simulink model "exemple4"  (R2021a)
settings: Solver=FixedStepDiscrete  StartTime=0.0  StopTime=0.1  RelTol=1e-3  EnableMultiTasking=on
values from neighbouring files (symbols this model uses):
  rep = reshape(a', 13*Ns, 1)'    [CalculREP.m]
  user = 1    [Launch_Sync.m]
libraries: dspsrcs4 x7, simulink x5, commfilt2 x4, dspsigops x3, dspswit3 x3, dspindex x2, commutil2 x1, simulink_extras x1
settings Model: Creator=sebastienroy  LastModifiedBy=antho
settings SolverCC: AlgebraicLoopSolver=TrustRegion
settings DataIOCC: InitialState=mod  LimitDataPoints=on  SaveFormat=Array  ReturnWorkspaceOutputs=off
settings OptimizationCC: LifeSpan=inf
settings DebuggingCC: UnderspecifiedInitializationDetection=Classic  MergeDetectMultiDrivingBlocksExec=none  SolverPrmCheckMsg=warning  StateNameClashWarn=warning  SFUnexpectedBacktrackingDiag=warning  SFNoUnconditionalDefaultTransitionDiag=warning  SFExecutionAtInitializationDiag=none  SFMachineParentedDataDiag=warning  ArithmeticOperatorsInVariantConditions=warning
settings HardwareCC: ProdBitPerPointer=32  ProdBitPerSizeT=32  ProdBitPerPtrDiffT=32  ProdLargestAtomicFloat=None  ProdIntDivRoundTo=Undefined  ProdEndianess=Unspecified  ProdWordSize=32  ProdHWDeviceType=32-bit Generic
settings ModelReferenceCC: PropagateSignalLabelsOutOfModel=off
settings SFSimCC: SimUseLocalCustomCode=off  CustomCodeUndefinedFunction=UseInterfaceOnly
settings RTWCC: RTWUseLocalCustomCode=off
settings CodeAppCC: StateflowObjectComments=on
settings GRTTargetCC: TargetLangStandard=C89/C90 (ANSI)
settings ConfigComp: CovMetricSettings=dw  CovSaveCumulativeToWorkspaceVar=on  CovSaveSingleToWorkspaceVar=on  CovExternalEMLEnable=off
settings SimscapeCC: SimscapeNormalizeSystem=off
settings ConfigurationSet: Description=SimMechanics 2G

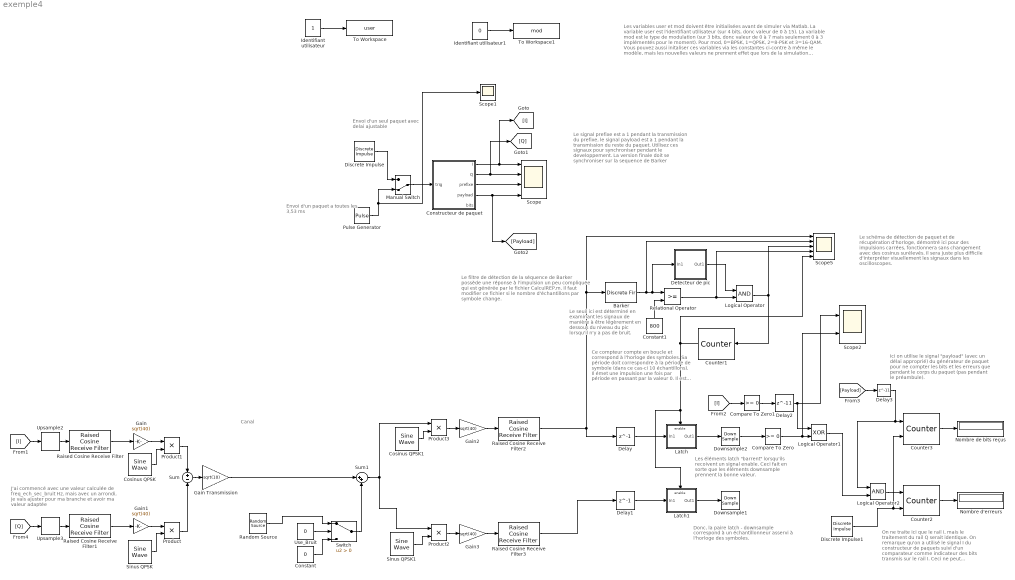
== system exemple4 ==
  note: Le filtre de détection de la séquence de Barker
      | possède une réponse à l'impulsion un peu
      | compliquée qui est générée par le fichier
      | CalculREP.m. Il faut modifier ce fichier si le nombre
      | d'échantillons par symbole change.
  note: Le schéma de détection de paquet et
      | de récupération d'horloge, démontré ici
      | pour des impulsions carrées, fonctionnera
      | sans changement avec des cosinus surélevés.
      | Il sera juste plus difficile d'interpréter visuellement
      | les signaux dans les oscilloscopes.
  note: On ne traite ici que le rail I, mais le
      | traitement du rail Q serait identique.
      | On remarque qu'on a utilisé le signal
      | I du constructeur de paquets suivi
      | d'un comparateur comme indicateur
      | des bits transmis sur le rail I. Ceci ne
      | peut fonctionner qu'en BPSK ou QPSK.
      | Dans le cas général, il faudrait utiliser la
      | sortie "bits" du générateur.
  note: Ici on utilise le signal "payload" (avec
      | un délai approprié) du générateur de
      | paquet pour ne compter les bits et les
      | erreurs que pendant le corps du paquet
      |  (pas pendant le préambule).
  note: Donc, la paire latch - downsample
      | correspond à un échantillonneur asservi
      | à l'horloge des symboles.
  note: Les éléments latch "barrent"
      | lorsqu'ils recoivent un signal enable.
      | Ceci fait en sorte que les éléments
      | downsample prennent la bonne valeur.
  note: Le seuil ici est déterminé
      | en examinant les signaux
      | de manière à être légèrement
      | en dessous du niveau du pic
      | lorsqu'il n'y a pas de bruit.
  note: Ce compteur compte en boucle et
      | correspond à l'horloge des symboles.
      | Sa période doit correspondre à
      | la période de symbole (dans ce
      | cas-ci 10 échantillons). Il émet
      | une impulsion une fois par
      | période en passant par la
      | valeur 0. Il est remis à zéro par
      | le pic de détection de début de paquet.
  note: Le signal prefixe est a 1 pendant
      | la transmission du prefixe, le signal payload
      | est a 1 pendant la transmission du reste du
      | paquet. Utilisez ces signaux pour synchroniser
      | pendant le developpement. La version finale
      | doit se synchroniser sur la sequence de Barker
  note: Les variables user et mod doivent être initialisées avant
      | de simuler via Matlab.
      | La variable user est l'identifiant utilisateur (sur 4 bits, donc valeur de 0 à 15).
      |
      | La variable mod est le type de modulation (sur 3 bits, donc valeur de 0 à 7
      | mais seulement 0 à 3 implémentés pour le moment). Pour mod, 0=BPSK,
      | 1=QPSK, 2=8-PSK et 3=16-QAM.
      |
      | Vous pouvez aussi initaliser ces variables via les constantes ci-contre à même
      | le modèle, mais les nouvelles valeurs ne prennent effet que lors de la simulation
      | suivante.
      |
      | Ces variables sont automatiquement incluses dans le préambule du paquet.
  note: Envoi d'un paquet
      | a toutes les 3,53 ms
  note: Envoi d'un seul
      | paquet avec delai
      | ajustable
  note: Canal
  note: J'ai commencé avec une valeur calculée de freq_ech_sec_bruit Hz, mais avec un arrondi, je vais ajuster pour ma branche et avoir ma valeur adaptée
  Barker : DiscreteFir  Coefficients=rep
  Compare To Zero : simulink/Logic and Bit Operations/Compare To Zero  relop=>=  OutDataTypeStr=boolean
  Compare To Zero1 : simulink/Logic and Bit Operations/Compare To Zero  relop=>=  OutDataTypeStr=boolean
  Constant : Constant  Value=0
  Constant1 : Constant  Value=800  SampleTime=-1
  Constructeur de paquet : Subsystem
  Cosinus QPSK : dspsrcs4/Sine Wave  Amplitude=1  Frequency=1.36e6  Phase=pi/2  SampleMode=Discrete  OutComplex=Real  CompMethod=Trigonometric fcn  TableSize=Speed  SampleTime=1/3400000  SamplesPerFrame=1  ResetState=Restart at time zero  OutputFrames=off  dataType=double  wordLen=16  udDataType=sfix(16)  fracBitsMode=Best precision  numFracBits=15  OutDataTypeStr=double  LastOutDataTypeStr=double
      settings: AttributesFormatString=|
      | Amplitude %<Amplitude>
      | Fréquence %<Frequency>
      | Phase %<Phase>
      | Sample Time %<SampleTime>
  Cosinus QPSK1 : dspsrcs4/Sine Wave  Amplitude=1  Frequency=1.36e6  Phase=pi/2  SampleMode=Discrete  OutComplex=Real  CompMethod=Trigonometric fcn  TableSize=Speed  SampleTime=1/3400000  SamplesPerFrame=1  ResetState=Restart at time zero  OutputFrames=off  dataType=double  wordLen=16  udDataType=sfix(16)  fracBitsMode=Best precision  numFracBits=15  OutDataTypeStr=double  LastOutDataTypeStr=double
      settings: AttributesFormatString=|
      | Amplitude %<Amplitude>
      | Fréquence %<Frequency>
      | Phase %<Phase>
      | Sample Time %<SampleTime>
  Counter1 : dspswit3/Counter  Direction=Up  CountEvent=Free running  CounterSize=User defined  MaxCount=9  InitialCount=0  Output=Hit  HitValue=0  ResetInput=on  SamplesPerFrame=1  Ts=-1  CntDtype=double  HitDtype=Logical
  Counter2 : dspswit3/Counter  Direction=Up  CountEvent=Non-zero sample  CounterSize=32 bits  MaxCount=255  InitialCount=0  Output=Count  HitValue=32  ResetInput=on  SamplesPerFrame=1  Ts=1/10000  CntDtype=double  HitDtype=Logical
  Counter3 : dspswit3/Counter  Direction=Up  CountEvent=Non-zero sample  CounterSize=32 bits  MaxCount=255  InitialCount=0  Output=Count  HitValue=32  ResetInput=on  SamplesPerFrame=1  Ts=1/10000  CntDtype=double  HitDtype=Logical
  Delay : Delay  DelayLength=1  InitialCondition=0
  Delay1 : Delay  DelayLength=1  InitialCondition=0
  Delay2 : Delay  DelayLength=11  InitialCondition=0
  Delay3 : Delay  DelayLength=11  InitialCondition=0
  Detecteur de pic : Subsystem
  Discrete Impulse : dspsrcs4/Discrete  Impulse  Delay=5  SampleTime=1/85000  FrameSample=1  OutputFrames=on  dataType=double  isSigned=on  wordLen=16  udDataType=sfix(16)  fracBitsMode=Best precision  numFracBits=15  OutDataTypeStr=double  LastOutDataTypeStr=double
  Discrete Impulse1 : dspsrcs4/Discrete  Impulse  Delay=6  SampleTime=1/85000  FrameSample=1  OutputFrames=on  dataType=double  isSigned=on  wordLen=16  udDataType=sfix(16)  fracBitsMode=Best precision  numFracBits=15  OutDataTypeStr=double  LastOutDataTypeStr=double
  Downsample1 : DownSample  N=40  RateOptions=Allow multirate processing
  Downsample2 : DownSample  N=40  RateOptions=Allow multirate processing
  Gain{,1..3} (4 alike) : Gain  Gain=sqrt(40)
  Gain Transmission : Gain  Gain=sqrt(10)
  Identifiant utilisateur : Constant  VectorParams1D=off
  Identifiant utilisateur1 : Constant  Value=0  VectorParams1D=off
  Latch : Subsystem  TreatAsAtomicUnit=on
  Latch1 : Subsystem  TreatAsAtomicUnit=on
  Logical Operator : Logic  AllPortsSameDT=off  OutDataTypeStr=boolean
  Logical Operator1 : Logic  Operator=XOR  AllPortsSameDT=off  OutDataTypeStr=boolean
  Logical Operator2 : Logic  AllPortsSameDT=off  OutDataTypeStr=boolean
  Manual Switch : ManualSwitch  CurrentSetting=0
  Nombre d'erreurs : Display
  Nombre de bits reçus : Display
  Product{,1..3} (4 alike) : Product
  Pulse Generator : DiscretePulseGenerator  Period=300  SampleTime=1/85000
  Raised Cosine Receive Filter : commfilt2/Raised Cosine Receive Filter  filtType=Square root  R=0.12  filtSpan=10  N=40  downFactor=1  downOffset=0  filterGain=1  RateOptions=Allow multirate processing  framing=Mute  checkCoeff=off  variableName=rcRxFilt  currentFiltSpan=10  D=5  inputOffset=0  sampMode=Mute  saveAsFlag=0  rateMode=Downsampling  checkGain=Normalized  launchFVT=on  roundingMode=Floor  overflowMode=off  coeffDataTypeStr=Inherit: Same word length as input  coeffMin=[]  coeffMax=[]  coeffLastDataTypeStr=Inherit: Same word length as input  accumDataTypeStr=Inherit: Same as product output  accumLastDataTypeStr=Inherit: Same as product output  outputDataTypeStr=Inherit: Same as accumulator  outputMin=[]  outputMax=[]  outputLastDataTypeStr=Inherit: Same as accumulator
      settings: AttributesFormatString=|
      | Type : %<filtType>
      | r : %<R>
      | Span in symb : %<filtSpan>
      | Gain : %<filterGain>
      | Input Samples per symb : 40
  Raised Cosine Receive Filter1 : commfilt2/Raised Cosine Receive Filter  filtType=Square root  R=0.12  filtSpan=10  N=40  downFactor=1  downOffset=0  filterGain=1  RateOptions=Allow multirate processing  framing=Mute  checkCoeff=off  variableName=rcRxFilt1  currentFiltSpan=10  D=5  inputOffset=0  sampMode=Mute  saveAsFlag=0  rateMode=Downsampling  checkGain=Normalized  launchFVT=on  roundingMode=Floor  overflowMode=off  coeffDataTypeStr=Inherit: Same word length as input  coeffMin=[]  coeffMax=[]  coeffLastDataTypeStr=Inherit: Same word length as input  accumDataTypeStr=Inherit: Same as product output  accumLastDataTypeStr=Inherit: Same as product output  outputDataTypeStr=Inherit: Same as accumulator  outputMin=[]  outputMax=[]  outputLastDataTypeStr=Inherit: Same as accumulator
      settings: AttributesFormatString=|
      | Type : %<filtType>
      | r : %<R>
      | Span in symb : %<filtSpan>
      | Gain : %<filterGain>
      | Input Samples per symb : 40
  Raised Cosine Receive Filter2 : commfilt2/Raised Cosine Receive Filter  filtType=Square root  R=0.12  filtSpan=10  N=40  downFactor=1  downOffset=0  filterGain=1  RateOptions=Allow multirate processing  framing=Mute  checkCoeff=off  variableName=rcRxFilt2  currentFiltSpan=10  D=5  inputOffset=0  sampMode=Mute  saveAsFlag=0  rateMode=Downsampling  checkGain=Normalized  launchFVT=on  roundingMode=Floor  overflowMode=off  coeffDataTypeStr=Inherit: Same word length as input  coeffMin=[]  coeffMax=[]  coeffLastDataTypeStr=Inherit: Same word length as input  accumDataTypeStr=Inherit: Same as product output  accumLastDataTypeStr=Inherit: Same as product output  outputDataTypeStr=Inherit: Same as accumulator  outputMin=[]  outputMax=[]  outputLastDataTypeStr=Inherit: Same as accumulator
      settings: AttributesFormatString=|
      | Type : %<filtType>
      | r : %<R>
      | Span in symb : %<filtSpan>
      | Gain : %<filterGain>
      | Input Samples per symb : 40
  Raised Cosine Receive Filter3 : commfilt2/Raised Cosine Receive Filter  filtType=Square root  R=0.12  filtSpan=10  N=40  downFactor=1  downOffset=0  filterGain=1  RateOptions=Allow multirate processing  framing=Mute  checkCoeff=off  variableName=rcRxFilt3  currentFiltSpan=10  D=5  inputOffset=0  sampMode=Mute  saveAsFlag=0  rateMode=Downsampling  checkGain=Normalized  launchFVT=on  roundingMode=Floor  overflowMode=off  coeffDataTypeStr=Inherit: Same word length as input  coeffMin=[]  coeffMax=[]  coeffLastDataTypeStr=Inherit: Same word length as input  accumDataTypeStr=Inherit: Same as product output  accumLastDataTypeStr=Inherit: Same as product output  outputDataTypeStr=Inherit: Same as accumulator  outputMin=[]  outputMax=[]  outputLastDataTypeStr=Inherit: Same as accumulator
      settings: AttributesFormatString=|
      | Type : %<filtType>
      | r : %<R>
      | Span in symb : %<filtSpan>
      | Gain : %<filterGain>
      | Input Samples per symb : 40
  Random Source : dspsrcs4/Random Source  SrcType=Gaussian  NormMethod=Ziggurat  CltLength=12  MinVal=0  MaxVal=1  MeanVal=0  VarVal=37.8072  RepMode=Not repeatable  rawSeed=1  IsInherit=off  SampMode=Discrete  SampTime=1/3.4e6  SampFrame=1  DataType=Double  OutComplex=Real  OutputFrames=off
      settings: AttributesFormatString=|
      | Sample Rate : 1/3.4e6 Hz
      | Variance : 37.8072 W
  Relational Operator : RelationalOperator  OutDataTypeStr=boolean  RndMeth=Nearest
  Scope : Scope  NumInputPorts=4
  Scope1 : Scope
  Scope2 : Scope  NumInputPorts=2
  Scope5 : Scope  NumInputPorts=5
  Sinus QPSK : dspsrcs4/Sine Wave  Amplitude=1  Frequency=1.36e6  Phase=0  SampleMode=Discrete  OutComplex=Real  CompMethod=Trigonometric fcn  TableSize=Speed  SampleTime=1/3400000  SamplesPerFrame=1  ResetState=Restart at time zero  OutputFrames=off  dataType=double  wordLen=16  udDataType=sfix(16)  fracBitsMode=Best precision  numFracBits=15  OutDataTypeStr=double  LastOutDataTypeStr=double
      settings: AttributesFormatString=|
      | Amplitude %<Amplitude>
      | Fréquence %<Frequency>
      | Phase %<Phase>
      | Sample Time %<SampleTime>
  Sinus QPSK1 : dspsrcs4/Sine Wave  Amplitude=-1  Frequency=1.36e6  Phase=0  SampleMode=Discrete  OutComplex=Real  CompMethod=Trigonometric fcn  TableSize=Speed  SampleTime=1/3400000  SamplesPerFrame=1  ResetState=Restart at time zero  OutputFrames=off  dataType=double  wordLen=16  udDataType=sfix(16)  fracBitsMode=Best precision  numFracBits=15  OutDataTypeStr=double  LastOutDataTypeStr=double
      settings: AttributesFormatString=|
      | Amplitude %<Amplitude>
      | Fréquence %<Frequency>
      | Phase %<Phase>
      | Sample Time %<SampleTime>
  Sum : Sum  Inputs=+|-
  Sum1 : Sum  Inputs=|++
  Switch : Switch  Criteria=u2 > Threshold
  To Workspace : ToWorkspace  VariableName=user  SampleTime=-1
      settings: Save2DSignal=2-D array (concatenate along first dimension)
  To Workspace1 : ToWorkspace  VariableName=mod  SampleTime=-1
      settings: Save2DSignal=2-D array (concatenate along first dimension)
  Upsample2 : dspsigops/Upsample  N=40  phase=0  RateOptions=Allow multirate processing  ic=0  mode=Unused parameter value
  Upsample3 : dspsigops/Upsample  N=40  phase=0  RateOptions=Allow multirate processing  ic=0  mode=Unused parameter value
  Use_Bruit : Constant  Value=0
  wires:
  Identifiant utilisateur/1 -> To Workspace/1
  Identifiant utilisateur1/1 -> To Workspace1/1
  Constructeur de paquet/3(prefixe) -> Scope/3
  Constructeur de paquet/1(I) -> [I], Scope/1
  Constructeur de paquet/4(payload) -> [Payload], Scope/4
  Constructeur de paquet/2(Q) -> Scope/2, [Q]
  Discrete Impulse/1 -> Manual Switch/1
  Manual Switch/1 -> Constructeur de paquet/1(trig)
  Pulse Generator/1 -> Scope1/1, Manual Switch/2
  Barker/1 -> Scope5/2, Detecteur de pic/1(In1), Relational Operator/1
  Constant1/1 -> Relational Operator/2
  Relational Operator/1 -> Logical Operator/2, Scope5/4
  Detecteur de pic/1(Out1) -> Logical Operator/1
  Logical Operator/1 -> Counter1/1, Scope5/3
  Latch/1(Out1) -> Downsample2/1
  Raised Cosine Receive Filter2/1 -> Delay/1, Barker/1, Scope5/1
  Latch1/1(Out1) -> Downsample1/1
  Raised Cosine Receive Filter3/1 -> Delay1/1
  Downsample2/1 -> Compare To Zero/1
  Counter1/1 -> Scope5/5, Latch1/Enable, Latch/Enable
  Delay/1 -> Latch/1(In1)
  Delay1/1 -> Latch1/1(In1)
  Compare To Zero/1 -> Scope2/2, Logical Operator1/2
  Delay2/1 -> Scope2/1, Logical Operator1/1
  Counter3/1 -> Nombre de bits reçus/1
  Counter2/1 -> Nombre d'erreurs/1
  Logical Operator2/1 -> Counter2/1
  [Payload] -> Delay3/1
  Delay3/1 -> Logical Operator2/1, Counter3/1
  Logical Operator1/1 -> Logical Operator2/2
  Discrete Impulse1/1 -> Counter3/2, Counter2/2
  [I] -> Compare To Zero1/1
  Compare To Zero1/1 -> Delay2/1
  Product2/1 -> Gain3/1
  Product1/1 -> Sum/1
  Random Source/1 -> Switch/1
  Use_Bruit/1 -> Switch/2
  Cosinus QPSK1/1 -> Product3/2
  Gain2/1 -> Raised Cosine Receive Filter2/1
  Gain3/1 -> Raised Cosine Receive Filter3/1
  Constant/1 -> Switch/3
  Upsample3/1 -> Raised Cosine Receive Filter1/1
  Gain1/1 -> Product/1
  Raised Cosine Receive Filter1/1 -> Gain1/1
  Switch/1 -> Sum1/2
  Raised Cosine Receive Filter/1 -> Gain/1
  Gain/1 -> Product1/1
  Product3/1 -> Gain2/1
  Sum/1 -> Gain Transmission/1
  Cosinus QPSK/1 -> Product1/2
  [Q] -> Upsample3/1
  Upsample2/1 -> Raised Cosine Receive Filter/1
  Product/1 -> Sum/2
  [I] -> Upsample2/1
  Sinus QPSK1/1 -> Product2/2
  Sinus QPSK/1 -> Product/2
  Gain Transmission/1 -> Sum1/1
  Sum1/1 -> Product2/1, Product3/1

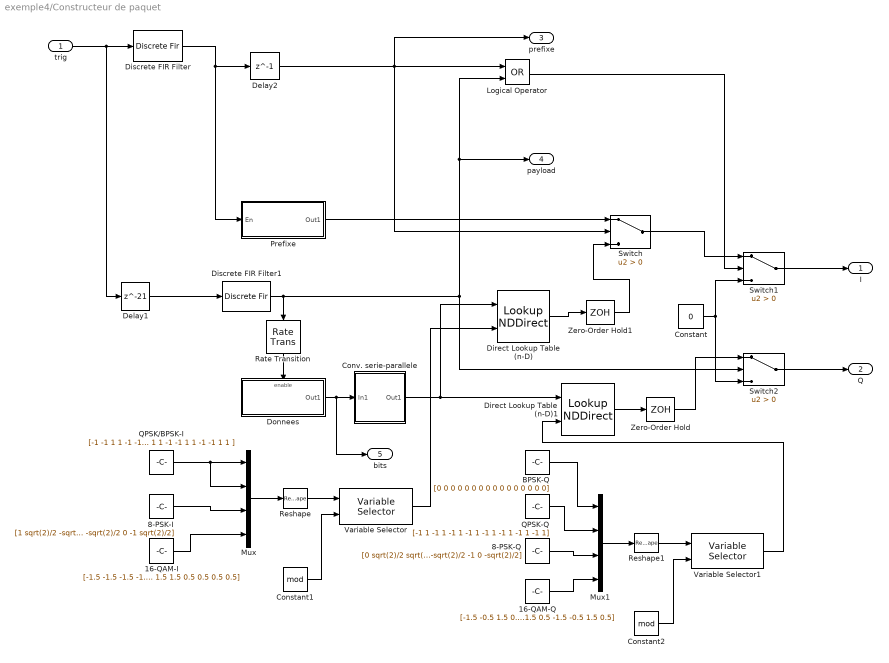
== system exemple4/Constructeur de paquet ==
  trig : Inport
  16-QAM-I : Constant  Value=[-1.5 -1.5 -1.5 -1.5 -0.5 -0.5 -0.5 -0.5 1.5 1.5 1.5 1.5 0.5 0.5 0.5 0.5]
  16-QAM-Q : Constant  Value=[-1.5 -0.5 1.5 0.5 -1.5 -0.5 1.5 0.5 -1.5 -0.5 1.5 0.5 -1.5 -0.5 1.5 0.5]
  8-PSK-I : Constant  Value=[1 sqrt(2)/2 -sqrt(2)/2 0 -sqrt(2)/2 0 -1 sqrt(2)/2 1 sqrt(2)/2 -sqrt(2)/2 0 -sqrt(2)/2 0 -1 sqrt(2)/2]
  8-PSK-Q : Constant  Value=[0 sqrt(2)/2 sqrt(2)/2 1 -sqrt(2)/2 -1 0 -sqrt(2)/2 0 sqrt(2)/2 sqrt(2)/2 1 -sqrt(2)/2 -1 0 -sqrt(2)/2]
  BPSK-Q : Constant  Value=[0 0 0 0 0 0 0 0 0 0 0 0 0 0 0 0]
  Constant : Constant  Value=0
  Constant1 : Constant  Value=mod
  Constant2 : Constant  Value=mod
  Conv. serie-parallele : Subsystem
  Delay1 : Delay  DelayLength=21
  Delay2 : Delay  DelayLength=1
  Direct Lookup Table (n-D) : LookupNDDirect  NumberOfTableDimensions=1  TableIsInput=on  Table=[0 2 3 2]
  Direct Lookup Table (n-D)1 : LookupNDDirect  NumberOfTableDimensions=1  TableIsInput=on  Table=[0 2 3 2]
  Discrete FIR Filter : DiscreteFir  Coefficients=ones(1,20)
  Discrete FIR Filter1 : DiscreteFir  Coefficients=ones(1,128)
  Donnees : Subsystem  TreatAsAtomicUnit=on
  Logical Operator : Logic  Operator=OR  AllPortsSameDT=off  OutDataTypeStr=boolean
  Mux : Mux
  Mux1 : Mux
  "Prefixe " : Subsystem  TreatAsAtomicUnit=on
  QPSK-Q : Constant  Value=[-1 1 -1 1 -1 1 -1 1 -1 1 -1 1 -1 1 -1 1]
  QPSK/BPSK-I : Constant  Value=[-1 -1 1 1 -1 -1 1 1 -1 -1 1 1 -1 -1 1 1 ]
  Rate Transition : RateTransition
  Reshape : Reshape  OutputDimensionality=Customize  OutputDimensions=[16,4]
  Reshape1 : Reshape  OutputDimensionality=Customize  OutputDimensions=[16,4]
  Switch : Switch  Criteria=u2 > Threshold
  Switch1 : Switch  Criteria=u2 > Threshold
  Switch2 : Switch  Criteria=u2 > Threshold
  Variable Selector : dspindex/Variable Selector  NumInputs=1  rowsOrCols=Columns  IdxMode=Variable  Elements=[1 3]  ZerOneIdxMode=Zero-based  errmode=Clip Index  FillMode=on  FillValues=0
  Variable Selector1 : dspindex/Variable Selector  NumInputs=1  rowsOrCols=Columns  IdxMode=Variable  Elements=[1 3]  ZerOneIdxMode=Zero-based  errmode=Clip Index  FillMode=on  FillValues=0
  Zero-Order Hold : ZeroOrderHold  SampleTime=1/85000
  Zero-Order Hold1 : ZeroOrderHold  SampleTime=1/85000
  I : Outport  VectorParamsAs1DForOutWhenUnconnected=off
  Q : Outport  Port=2  VectorParamsAs1DForOutWhenUnconnected=off
  prefixe : Outport  Port=3  VectorParamsAs1DForOutWhenUnconnected=off
  payload : Outport  Port=4  VectorParamsAs1DForOutWhenUnconnected=off
  bits : Outport  Port=5  VectorParamsAs1DForOutWhenUnconnected=off
  wires:
  "Prefixe "/1(Out1) -> Switch/1
  Switch2/1 -> Q/1
  Constant/1 -> Switch2/3, Switch1/3
  trig/1 -> Delay1/1, Discrete FIR Filter/1
  Delay1/1 -> Discrete FIR Filter1/1
  Switch/1 -> Switch1/1
  Logical Operator/1 -> Switch1/2
  Discrete FIR Filter/1 -> Delay2/1, "Prefixe "/1(En)
  Switch1/1 -> I/1
  Discrete FIR Filter1/1 -> Rate Transition/1, Switch2/2, payload/1, Logical Operator/2
  Rate Transition/1 -> Donnees/Enable
  Donnees/1(Out1) -> bits/1, Conv. serie-parallele/1(In1)
  Conv. serie-parallele/1(Out1) -> Direct Lookup Table (n-D)/1, Direct Lookup Table (n-D)1/1
  Direct Lookup Table (n-D)/1 -> Zero-Order Hold1/1
  Zero-Order Hold1/1 -> Switch/3
  Direct Lookup Table (n-D)1/1 -> Zero-Order Hold/1
  Zero-Order Hold/1 -> Switch2/1
  QPSK/BPSK-I/1 -> Mux/2, Mux/1
  16-QAM-I/1 -> Mux/4
  8-PSK-I/1 -> Mux/3
  Variable Selector/1 -> Direct Lookup Table (n-D)/2
  Mux/1 -> Reshape/1
  Constant1/1 -> Variable Selector/2
  Reshape/1 -> Variable Selector/1
  Reshape1/1 -> Variable Selector1/1
  Constant2/1 -> Variable Selector1/2
  Mux1/1 -> Reshape1/1
  BPSK-Q/1 -> Mux1/1
  QPSK-Q/1 -> Mux1/2
  16-QAM-Q/1 -> Mux1/4
  8-PSK-Q/1 -> Mux1/3
  Variable Selector1/1 -> Direct Lookup Table (n-D)1/2
  Delay2/1 -> prefixe/1, Switch/2, Logical Operator/1

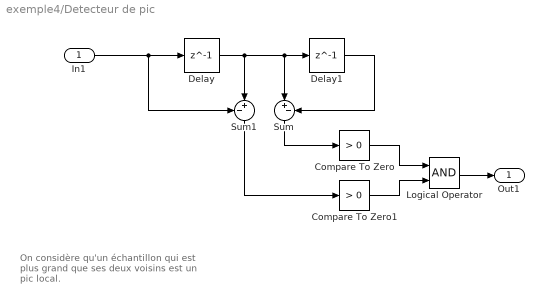
== system exemple4/Detecteur de pic ==
  note: On considère qu'un échantillon qui
      | est plus grand que ses deux voisins
      | est un pic local.
  In1 : Inport
  Compare To Zero : simulink/Logic and Bit Operations/Compare To Zero  relop=>  OutDataTypeStr=boolean
  Compare To Zero1 : simulink/Logic and Bit Operations/Compare To Zero  relop=>  OutDataTypeStr=boolean
  Delay : Delay  DelayLength=1  InitialCondition=0
  Delay1 : Delay  DelayLength=1  InitialCondition=0
  Logical Operator : Logic  AllPortsSameDT=off  OutDataTypeStr=boolean
  Sum : Sum  Inputs=|+-
  Sum1 : Sum  Inputs=-+|
  Out1 : Outport
  wires:
  In1/1 -> Sum1/1, Delay/1
  Delay1/1 -> Sum/2
  Delay/1 -> Sum1/2, Sum/1, Delay1/1
  Sum/1 -> Compare To Zero/1
  Sum1/1 -> Compare To Zero1/1
  Compare To Zero/1 -> Logical Operator/1
  Compare To Zero1/1 -> Logical Operator/2
  Logical Operator/1 -> Out1/1

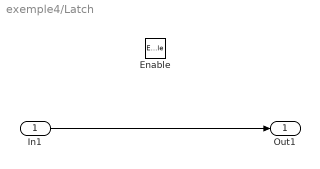
== system exemple4/Latch ==
  In1 : Inport
  Enable : EnablePort
  Out1 : Outport  VectorParamsAs1DForOutWhenUnconnected=off
  wires:
  In1/1 -> Out1/1

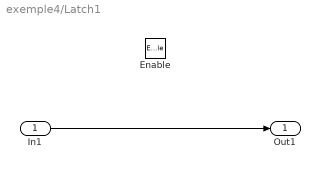
== system exemple4/Latch1 ==
  In1 : Inport
  Enable : EnablePort
  Out1 : Outport  VectorParamsAs1DForOutWhenUnconnected=off
  wires:
  In1/1 -> Out1/1

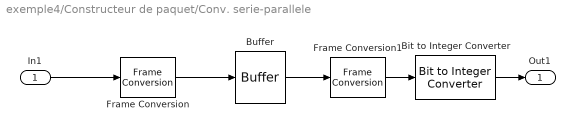
== system exemple4/Constructeur de paquet/Conv. serie-parallele ==
  In1 : Inport
  Bit to Integer Converter : commutil2/Bit to Integer Converter  nbits=4  bitOrder=MSB first  signedOutputValues=Unsigned  outDtype=Inherit via internal rule  outDtypeSigned=Inherit via internal rule
  Buffer : Buffer  N=4
  Frame Conversion : FrameConversion
  Frame Conversion1 : FrameConversion  OutFrame=Sample-based
  Out1 : Outport  VectorParamsAs1DForOutWhenUnconnected=off
  wires:
  Buffer/1 -> Frame Conversion1/1
  In1/1 -> Frame Conversion/1
  Frame Conversion/1 -> Buffer/1
  Frame Conversion1/1 -> Bit to Integer Converter/1
  Bit to Integer Converter/1 -> Out1/1

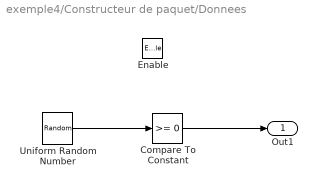
== system exemple4/Constructeur de paquet/Donnees ==
  Enable : EnablePort
  Compare To Constant : simulink/Logic and Bit Operations/Compare To Constant  relop=>=  const=0  OutDataTypeStr=boolean
      link override Compare: Operator=>=  OutDataTypeStr=boolean
  Uniform Random Number : UniformRandomNumber  Seed=17  SampleTime=1/340000
  Out1 : Outport  VectorParamsAs1DForOutWhenUnconnected=off
  wires:
  Uniform Random Number/1 -> Compare To Constant/1
  Compare To Constant/1 -> Out1/1

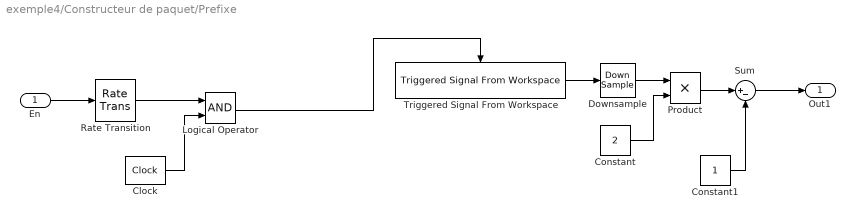
== system exemple4/Constructeur de paquet/Prefixe  ==
  En : Inport
  Clock : simulink_extras/Flip Flops/Clock  period=1/85000
  Constant : Constant  Value=2
  Constant1 : Constant
  Downsample : DownSample  RateOptions=Allow multirate processing
  Logical Operator : Logic  AllPortsSameDT=off  OutDataTypeStr=boolean
  Product : Product
  Rate Transition : RateTransition  OutPortSampleTime=1/170000
  Sum : Sum  Inputs=|+-
  Triggered Signal From Workspace : dspsigops/Triggered Signal From Workspace  Signal=[1 1 1 1 1 0 0 1 1 0 1 0 1 fliplr(de2bi(user,3)) fliplr(de2bi(mod,4))]  TriggerType=Rising edge  ic=0  SamplesPerFrame=1  OutputAfterFinalValue=Cyclic repetition  OutputFrames=on
      settings: SourceProductBaseCode=DS
  Out1 : Outport  VectorParamsAs1DForOutWhenUnconnected=off
  wires:
  Triggered Signal From Workspace/1 -> Downsample/1
  Clock/1 -> Logical Operator/2
  En/1 -> Rate Transition/1
  Logical Operator/1 -> Triggered Signal From Workspace/Trigger
  Rate Transition/1 -> Logical Operator/1
  Downsample/1 -> Product/1
  Constant/1 -> Product/2
  Product/1 -> Sum/1
  Constant1/1 -> Sum/2
  Sum/1 -> Out1/1
